simulink model "PropulsionPlant"  (R2022b)
settings: Solver=VariableStepAuto  StartTime=0.0  StopTime=10.0  RelTol=1e-3
undefined symbols (not defined in the file or in its folder): Bat, ESC, fan, LookUp, motor
settings Model: Creator=User  LastModifiedBy=User

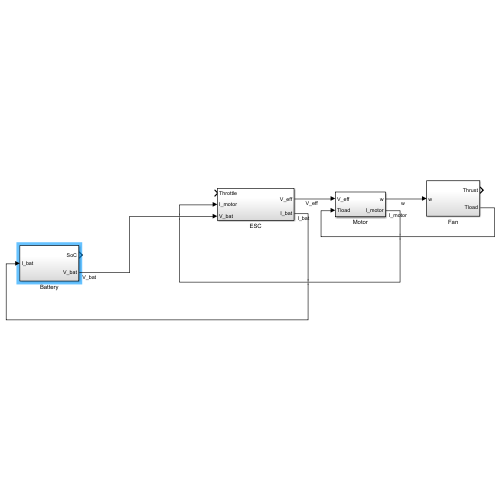
[thumbnail: Simulink's stored preview of the top-level diagram]
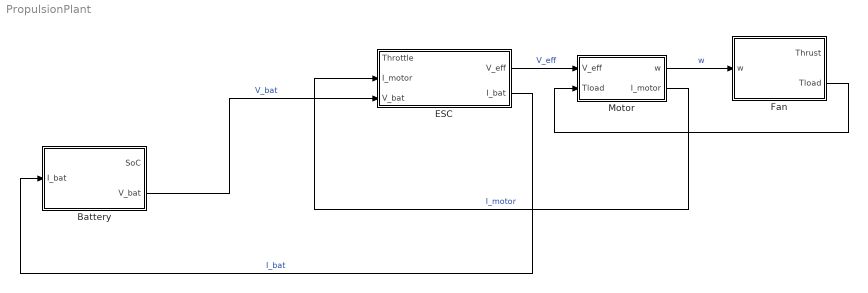
== system PropulsionPlant ==
  Battery : Subsystem
  ESC : Subsystem
  Fan : Subsystem
  Motor : Subsystem
  wires:
  Fan/2(Tload) -> Motor/2(Tload)
  ESC/1(V_eff) -> Motor/1(V_eff)  "V_eff"
  Motor/2(I_motor) -> ESC/2(I_motor)  "I_motor"
  Motor/1(w) -> Fan/1(w)  "w"
  ESC/2(I_bat) -> Battery/1(I_bat)  "I_bat"
  Battery/2(V_bat) -> ESC/3(V_bat)  "V_bat"

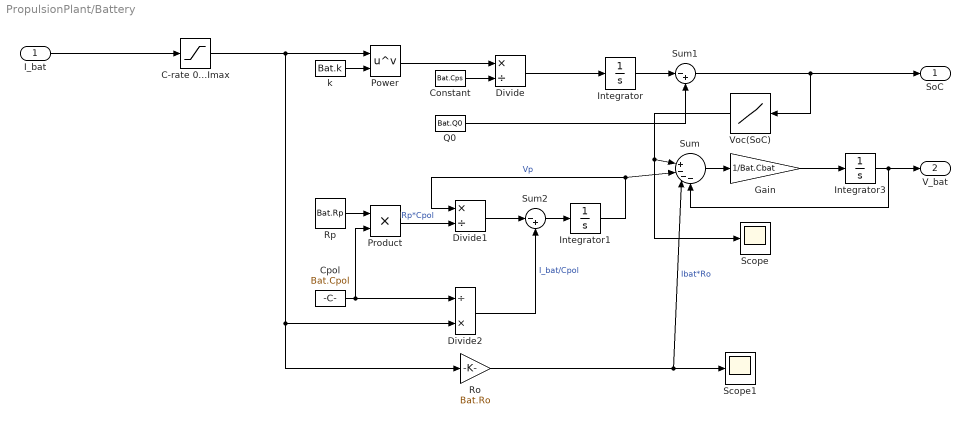
== system PropulsionPlant/Battery ==
  I_bat : Inport
  C-rate 0...Imax : Saturate  UpperLimit=Bat.Imax  LowerLimit=0
  Constant : Constant  Value=Bat.Cps
  Cpol : Constant  Value=Bat.Cpol
  Divide : Product  Inputs=*/
  Divide1 : Product  Inputs=*/
  Divide2 : Product  Inputs=/*
  Gain : Gain  Gain=1/Bat.Cbat
  Integrator : Integrator
  Integrator1 : Integrator
  Integrator3 : Integrator  InitialCondition=Bat.Vcell*Bat.ncell
  Power : Math  Operator=pow
  Product : Product
  Q0 : Constant  Value=Bat.Q0
  Ro : Gain  Gain=Bat.Ro
  Rp : Constant  Value=Bat.Rp
  Scope : Scope
  Scope1 : Scope
  Sum : Sum  Inputs=||+---
  Sum1 : Sum  Inputs=|-+
  Sum2 : Sum  Inputs=|-+
  Voc(SoC) : Lookup_n-D  NumberOfTableDimensions=1  BreakpointsForDimension1=LookUp.SoC  Table=LookUp.Volts  InternalRulePriority=Speed  RndMeth=Simplest
  k : Constant  Value=Bat.k
  SoC : Outport
  V_bat : Outport  Port=2
  wires:
  Integrator1/1 -> Divide1/1, Sum/2  "Vp"
  Sum2/1 -> Integrator1/1
  Product/1 -> Divide1/2  "Rp*Cpol"
  Q0/1 -> Sum1/2
  Cpol/1 -> Divide2/1, Product/2
  Voc(SoC)/1 -> Scope/1, Sum/1
  Rp/1 -> Product/1
  Power/1 -> Divide/1
  Constant/1 -> Divide/2
  k/1 -> Power/2
  Sum/1 -> Gain/1
  I_bat/1 -> C-rate 0...Imax/1
  Integrator/1 -> Sum1/1
  Sum1/1 -> Voc(SoC)/1, SoC/1
  Divide1/1 -> Sum2/1
  Divide2/1 -> Sum2/2  "I_bat/Cpol"
  Ro/1 -> Sum/3, Scope1/1  "Ibat*Ro"
  Divide/1 -> Integrator/1
  C-rate 0...Imax/1 -> Ro/1, Divide2/2, Power/1
  Integrator3/1 -> Sum/4, V_bat/1
  Gain/1 -> Integrator3/1

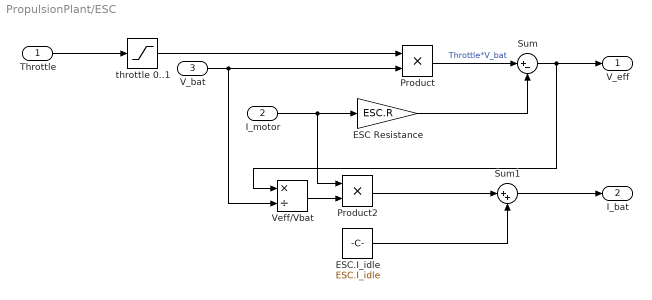
== system PropulsionPlant/ESC ==
  Throttle : Inport
  I_motor : Inport  Port=2
  V_bat : Inport  Port=3
  ESC Resistance : Gain  Gain=ESC.R
  ESC.I_idle : Constant  Value=ESC.I_idle
  Product : Product
  Product2 : Product
  Sum : Sum  Inputs=|+-
  Sum1 : Sum  Inputs=|++
  Veff/Vbat : Product  Inputs=*/
  throttle 0..1 : Saturate  UpperLimit=1  LowerLimit=0
  V_eff : Outport
  I_bat : Outport  Port=2
  wires:
  Throttle/1 -> throttle 0..1/1
  V_bat/1 -> Product/2, Veff/Vbat/2
  Product/1 -> Sum/1  "Throttle*V_bat"
  Sum1/1 -> I_bat/1
  ESC Resistance/1 -> Sum/2
  Sum/1 -> V_eff/1, Veff/Vbat/1
  I_motor/1 -> ESC Resistance/1, Product2/1
  Veff/Vbat/1 -> Product2/2
  Product2/1 -> Sum1/1
  ESC.I_idle/1 -> Sum1/2
  throttle 0..1/1 -> Product/1

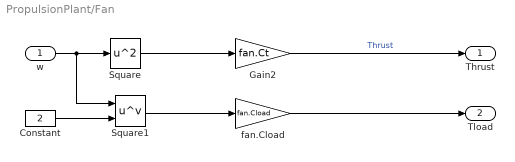
== system PropulsionPlant/Fan ==
  w : Inport
  Constant : Constant  Value=2
  Gain2 : Gain  Gain=fan.Ct
  Square : Math  Operator=square
  Square1 : Math  Operator=pow
  fan.Cload : Gain  Gain=fan.Cload
  Thrust : Outport
  Tload : Outport  Port=2
  wires:
  Square/1 -> Gain2/1
  Gain2/1 -> Thrust/1  "Thrust"
  w/1 -> Square1/1, Square/1
  Constant/1 -> Square1/2
  Square1/1 -> fan.Cload/1
  fan.Cload/1 -> Tload/1

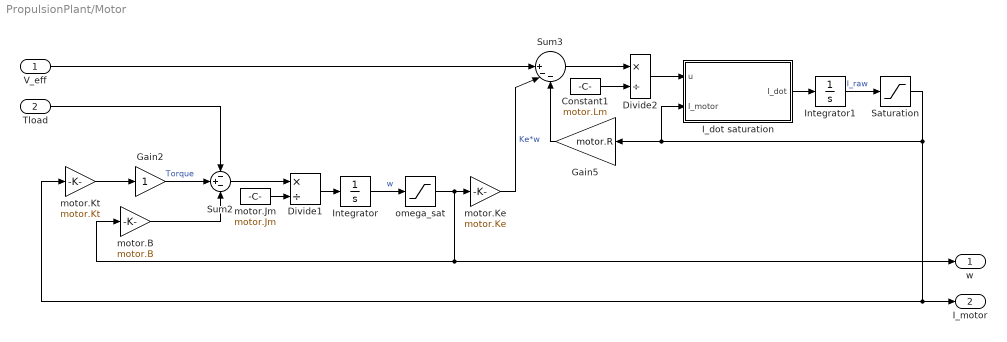
== system PropulsionPlant/Motor ==
  V_eff : Inport
  Tload : Inport  Port=2
  Constant1 : Constant  Value=motor.Lm
  Divide1 : Product  Inputs=*/
  Divide2 : Product  Inputs=*/
  Gain2 : Gain
  Gain5 : Gain  Gain=motor.R
  I_dot saturation : MATLAB Function  TreatAsAtomicUnit=on
  Integrator : Integrator
  Integrator1 : Integrator
  Saturation : Saturate  UpperLimit=motor.Imax  LowerLimit=-motor.Imax
  Sum2 : Sum  Inputs=-+-
  Sum3 : Sum  Inputs=||+--
  motor.B : Gain  Gain=motor.B
  motor.Jm : Constant  Value=motor.Jm
  motor.Ke : Gain  Gain=motor.Ke
  motor.Kt : Gain  Gain=motor.Kt
  omega_sat : Saturate  UpperLimit=motor.maxFreq  LowerLimit=0
  w : Outport
  I_motor : Outport  Port=2
  wires:
  motor.Jm/1 -> Divide1/2
  Divide1/1 -> Integrator/1
  motor.Kt/1 -> Gain2/1
  Integrator/1 -> omega_sat/1  "w"
  Constant1/1 -> Divide2/2
  motor.Ke/1 -> Sum3/2  "Ke*w"
  Integrator1/1 -> Saturation/1  "I_raw"
  V_eff/1 -> Sum3/1
  Gain2/1 -> Sum2/2  "Torque"
  Sum2/1 -> Divide1/1
  Tload/1 -> Sum2/1
  motor.B/1 -> Sum2/3
  Sum3/1 -> Divide2/1
  Gain5/1 -> Sum3/3
  Saturation/1 -> I_dot saturation/2(I_motor), Gain5/1, motor.Kt/1, I_motor/1
  Divide2/1 -> I_dot saturation/1(u)
  I_dot saturation/1(I_dot) -> Integrator1/1
  omega_sat/1 -> motor.B/1, w/1, motor.Ke/1

== matlab function PropulsionPlant/Motor/I_dot saturation ==
  data: u input; I_dot output; I_motor input
function I_dot = Idot(u, I_motor)

% parameters (define as mask parameters or globals)
I_max = 120;     % example
u_max = 1e6;     % A/s, numerical safety limit

% guard against NaN / Inf
if ~isfinite(u)
    I_dot = 0;
    return;
end

% limit derivative (ESC bandwidth / numerical safety)
u = max(min(u, u_max), -u_max);

% saturation detection (NOT at zero!)
sat = abs(I_motor) >= I_max;

% pushing further only if current is nonzero
push = (I_motor ~= 0) && (sign(u) == sign(I_motor));

if sat && push
    I_dot = 0;
else
    I_dot = u;
end
